simulink model "nl_cart_1"  (R2022a)
settings: Solver=ode45  StartTime=0.0  StopTime=5  MaxStep=0.001  MinStep=0.000001  RelTol=1e-3
values from neighbouring files (symbols this model uses):
  b = 0    [ex1.m]    (also in ex2.m = 1; ex3.m = 1; lab3es2_20230414.m = 1)
  dth0 = 0    [ex1.m]    (also in ex2.m; ex3.m)
  dx0 = 0.1    [ex1.m]    (also in ex2.m = 0; ex3.m = 0)
  g = 9.81    [ex1.m]    (also in ex2.m; ex3.m; lab3es2_20230414.m)
  Ie = I + m * l^2    (= 0.02603525)    [ex1.m]    (also in ex2.m; ex3.m; lab3es2_20230414.m = 0.026047)
  k = 10    [ex1.m]    (also in lab3es2_20230414.m)
  l = 0.305    [ex1.m]    (also in ex2.m; ex3.m; lab3es2_20230414.m)
  m = 0.21    [ex1.m]    (also in ex2.m; ex3.m; lab3es2_20230414.m)
  Me = M + m    (= 0.665)    [ex1.m]    (also in ex2.m; ex3.m; lab3es2_20230414.m)
  th0 = pi * 7 / 8    (= 2.74889357189)    [ex1.m]    (also in ex2.m = 0; ex3.m = 0)
  x0 = 1    [ex1.m]    (also in ex2.m = 0; ex3.m = 10)
settings Model: Creator=loren  LastModifiedBy=loren
settings DataIOCC: ReturnWorkspaceOutputs=off

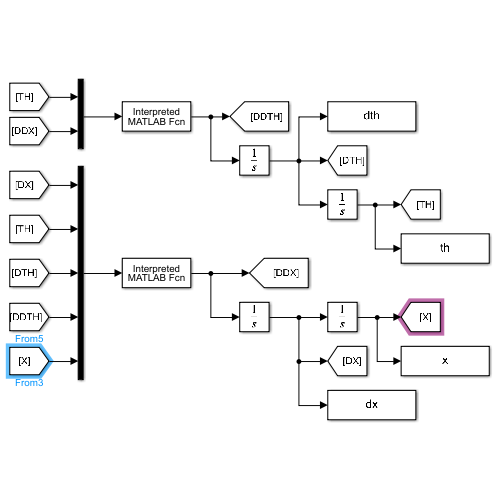
[thumbnail: Simulink's stored preview of the top-level diagram]
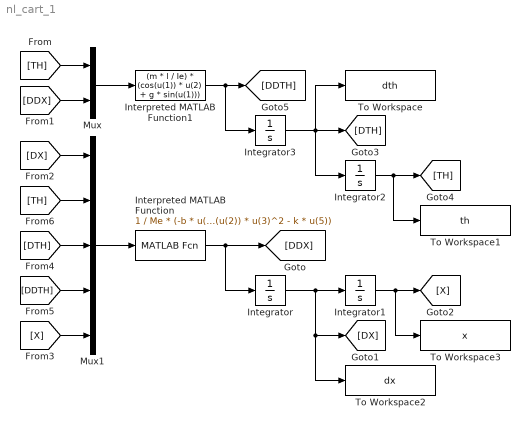
== system nl_cart_1 ==
  Integrator : Integrator  InitialCondition=dx0
  Integrator1 : Integrator  InitialCondition=x0
  Integrator2 : Integrator  InitialCondition=th0
  Integrator3 : Integrator  InitialCondition=dth0
  Interpreted MATLAB Function : MATLABFcn  MATLABFcn=1 / Me * (-b * u(1) + m * l * cos(u(2)) * u(4) - m * l * sin(u(2)) * u(3)^2 - k * u(5))  OutputDimensions=1
  Interpreted MATLAB Function1 : MATLABFcn  MATLABFcn=(m * l / Ie) * (cos(u(1)) * u(2) + g * sin(u(1)))  OutputDimensions=1
  Mux : Mux  Inputs=2
  Mux1 : Mux  Inputs=5
  To Workspace : ToWorkspace  VariableName=dth  SaveFormat=Timeseries  SampleTime=-1
  To Workspace1 : ToWorkspace  VariableName=th  SaveFormat=Timeseries  SampleTime=-1
  To Workspace2 : ToWorkspace  VariableName=dx  SaveFormat=Timeseries  SampleTime=-1
  To Workspace3 : ToWorkspace  VariableName=x  SaveFormat=Timeseries  SampleTime=-1
  wires:
  [TH] -> Mux/1
  [DDX] -> Mux/2
  Integrator2/1 -> To Workspace1/1, [TH]
  Integrator1/1 -> To Workspace3/1, [X]
  [TH] -> Mux1/2
  [DTH] -> Mux1/3
  Mux1/1 -> Interpreted MATLAB Function/1
  Mux/1 -> Interpreted MATLAB Function1/1
  [DX] -> Mux1/1
  [X] -> Mux1/5
  [DDTH] -> Mux1/4
  Integrator3/1 -> To Workspace/1, Integrator2/1, [DTH]
  Integrator/1 -> Integrator1/1, To Workspace2/1, [DX]
  Interpreted MATLAB Function/1 -> Integrator/1, [DDX]
  Interpreted MATLAB Function1/1 -> Integrator3/1, [DDTH]
